simulink library "Displays_Lib"  (Simulink 8.1)
settings: Solver=ode45  StartTime=0.0  StopTime=10.0  RelTol=1e-3
undefined symbols (not defined in the file): ending_column_index, ending_row_index, framebuffer_16x1, framebuffer_2x2, framebuffer_4x4, framebuffer_8x8, HEIGHT, hot, POS_X, POS_Y, starting_column_index, starting_row_index, WIDTH
libraries: dspmtrx3 x119, commutil2 x100, dspsnks4 x4
(part 2 of 2)

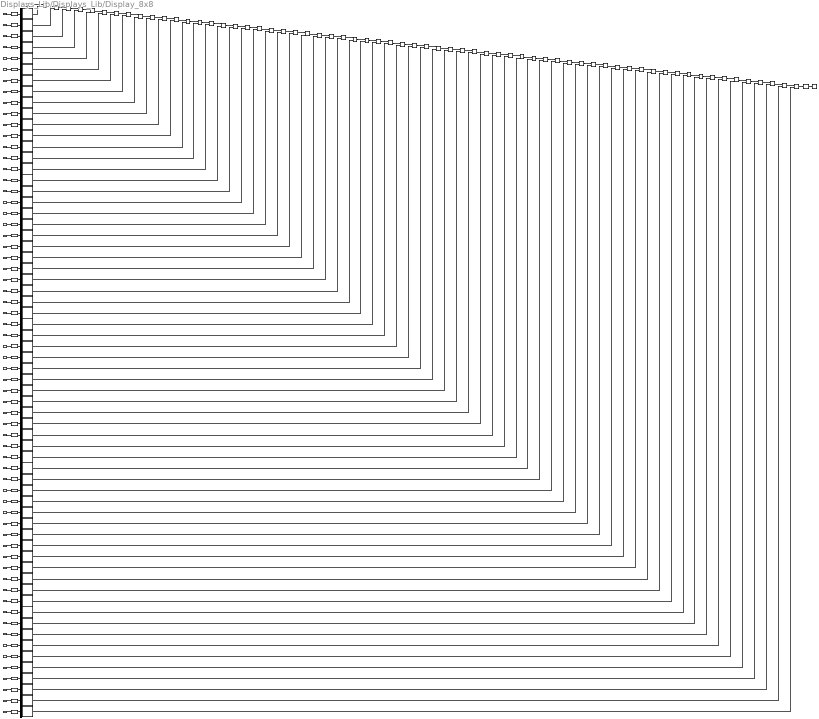
== system Displays_Lib/Displays_Lib/Display_8x8 ==
  Row1_Col1(8x1B) : Inport
  Row1_Col2(8x1B) : Inport  Port=2
  Row1_Col3(8x1B) : Inport  Port=3
  Row1_Col4(8x1B) : Inport  Port=4
  Row1_Col5(8x1B) : Inport  Port=5
  Row1_Col6(8x1B) : Inport  Port=6
  Row1_Col7(8x1B) : Inport  Port=7
  Row1_Col8(8x1B) : Inport  Port=8
  Row2_Col1(8x1B) : Inport  Port=9
  Row2_Col2(8x1B) : Inport  Port=10
  Row2_Col3(8x1B) : Inport  Port=11
  Row2_Col4(8x1B) : Inport  Port=12
  Row2_Col5(8x1B) : Inport  Port=13
  Row2_Col6(8x1B) : Inport  Port=14
  Row2_Col7(8x1B) : Inport  Port=15
  Row2_Col8(8x1B) : Inport  Port=16
  Row3_Col1(8x1B) : Inport  Port=17
  Row3_Col2(8x1B) : Inport  Port=18
  Row3_Col3(8x1B) : Inport  Port=19
  Row3_Col4(8x1B) : Inport  Port=20
  Row3_Col5(8x1B) : Inport  Port=21
  Row3_Col6(8x1B) : Inport  Port=22
  Row3_Col7(8x1B) : Inport  Port=23
  Row3_Col8(8x1B) : Inport  Port=24
  Row4_Col1(8x1B) : Inport  Port=25
  Row4_Col2(8x1B) : Inport  Port=26
  Row4_Col3(8x1B) : Inport  Port=27
  Row4_Col4(8x1B) : Inport  Port=28
  Row4_Col5(8x1B) : Inport  Port=29
  Row4_Col6(8x1B) : Inport  Port=30
  Row4_Col7(8x1B) : Inport  Port=31
  Row4_Col8(8x1B) : Inport  Port=32
  Row5_Col1(8x1B) : Inport  Port=33
  Row5_Col2(8x1B) : Inport  Port=34
  Row5_Col3(8x1B) : Inport  Port=35
  Row5_Col4(8x1B) : Inport  Port=36
  Row5_Col5(8x1B) : Inport  Port=37
  Row5_Col6(8x1B) : Inport  Port=38
  Row5_Col7(8x1B) : Inport  Port=39
  Row5_Col8(8x1B) : Inport  Port=40
  Row6_Col1(8x1B) : Inport  Port=41
  Row6_Col2(8x1B) : Inport  Port=42
  Row6_Col3(8x1B) : Inport  Port=43
  Row6_Col4(8x1B) : Inport  Port=44
  Row6_Col5(8x1B) : Inport  Port=45
  Row6_Col6(8x1B) : Inport  Port=46
  Row6_Col7(8x1B) : Inport  Port=47
  Row6_Col8(8x1B) : Inport  Port=48
  Row7_Col1(8x1B) : Inport  Port=49
  Row7_Col2(8x1B) : Inport  Port=50
  Row7_Col3(8x1B) : Inport  Port=51
  Row7_Col4(8x1B) : Inport  Port=52
  Row7_Col5(8x1B) : Inport  Port=53
  Row7_Col6(8x1B) : Inport  Port=54
  Row7_Col7(8x1B) : Inport  Port=55
  Row7_Col8(8x1B) : Inport  Port=56
  Row8_Col1(8x1B) : Inport  Port=57
  Row8_Col2(8x1B) : Inport  Port=58
  Row8_Col3(8x1B) : Inport  Port=59
  Row8_Col4(8x1B) : Inport  Port=60
  Row8_Col5(8x1B) : Inport  Port=61
  Row8_Col6(8x1B) : Inport  Port=62
  Row8_Col7(8x1B) : Inport  Port=63
  Row8_Col8(8x1B) : Inport  Port=64
  Constant1 : Constant  Value=framebuffer_8x8  OutDataTypeStr=uint8
  Demux{1..3,20..80} (64 alike) : Demux  Outputs=8
  Integer to Bit Converter{1..3,17,21..80} (64 alike) : commutil2/Integer to Bit Converter  nbits=8  signedInputValues=Unsigned  bitOrder=MSB first  outDtype=uint8
  Matrix Concatenate{1..4,21..80} (64 alike) : Concatenate  NumInputs=8  Mode=Multidimensional array  ConcatenateDimension=2
  Matrix Viewer3 : dspsnks4/Matrix Viewer  ImageParams=off  CMapStr=hot(256)  AxisColorbar=on  AxisParams=off  AxisOrigin=Upper left corner  XLabel=X-axis  YLabel=Y-axis  ZLabel=Z-axis  FigPos=[POS_X POS_Y-140 WIDTH HEIGHT]  AxisZoom=on
      settings: YMin=0  YMax=1.0
  Overwrite Values1 : dspmtrx3/Overwrite Values  OverWriteDiag=Submatrix  valFrom2ndIP=Second input port  ConstValue=0  RowSpan=Range of rows  RowStartMode=Index  RowStartIndex=starting_row_index(3)  RowEndMode=Index  RowEndIndex=ending_row_index(3)  ColSpan=Range of columns  ColStartMode=Index  ColStartIndex=starting_column_index(2)  ColEndMode=Index  ColEndIndex=ending_column_index(2)  DiagSpan=Range of elements  DiagStartMode=Index  DiagStartIndex=2  DiagEndMode=Index  DiagEndIndex=4
  Overwrite Values15 : dspmtrx3/Overwrite Values  OverWriteDiag=Submatrix  valFrom2ndIP=Second input port  ConstValue=0  RowSpan=Range of rows  RowStartMode=Index  RowStartIndex=starting_row_index(3)  RowEndMode=Index  RowEndIndex=ending_row_index(3)  ColSpan=Range of columns  ColStartMode=Index  ColStartIndex=starting_column_index(4)  ColEndMode=Index  ColEndIndex=ending_column_index(4)  DiagSpan=Range of elements  DiagStartMode=Index  DiagStartIndex=2  DiagEndMode=Index  DiagEndIndex=4
  Overwrite Values17 : dspmtrx3/Overwrite Values  OverWriteDiag=Submatrix  valFrom2ndIP=Second input port  ConstValue=0  RowSpan=Range of rows  RowStartMode=Index  RowStartIndex=starting_row_index(3)  RowEndMode=Index  RowEndIndex=ending_row_index(3)  ColSpan=Range of columns  ColStartMode=Index  ColStartIndex=starting_column_index(1)  ColEndMode=Index  ColEndIndex=ending_column_index(1)  DiagSpan=Range of elements  DiagStartMode=Index  DiagStartIndex=2  DiagEndMode=Index  DiagEndIndex=4
  Overwrite Values18 : dspmtrx3/Overwrite Values  OverWriteDiag=Submatrix  valFrom2ndIP=Second input port  ConstValue=0  RowSpan=Range of rows  RowStartMode=Index  RowStartIndex=starting_row_index(5)  RowEndMode=Index  RowEndIndex=ending_row_index(5)  ColSpan=Range of columns  ColStartMode=Index  ColStartIndex=starting_column_index(2)  ColEndMode=Index  ColEndIndex=ending_column_index(2)  DiagSpan=Range of elements  DiagStartMode=Index  DiagStartIndex=2  DiagEndMode=Index  DiagEndIndex=4
  Overwrite Values19 : dspmtrx3/Overwrite Values  OverWriteDiag=Submatrix  valFrom2ndIP=Second input port  ConstValue=0  RowSpan=Range of rows  RowStartMode=Index  RowStartIndex=starting_row_index(4)  RowEndMode=Index  RowEndIndex=ending_row_index(4)  ColSpan=Range of columns  ColStartMode=Index  ColStartIndex=starting_column_index(4)  ColEndMode=Index  ColEndIndex=ending_column_index(4)  DiagSpan=Range of elements  DiagStartMode=Index  DiagStartIndex=2  DiagEndMode=Index  DiagEndIndex=4
  Overwrite Values2 : dspmtrx3/Overwrite Values  OverWriteDiag=Submatrix  valFrom2ndIP=Second input port  ConstValue=0  RowSpan=Range of rows  RowStartMode=Index  RowStartIndex=starting_row_index(8)  RowEndMode=Index  RowEndIndex=ending_row_index(8)  ColSpan=Range of columns  ColStartMode=Index  ColStartIndex=starting_column_index(3)  ColEndMode=Index  ColEndIndex=ending_column_index(3)  DiagSpan=Range of elements  DiagStartMode=Index  DiagStartIndex=2  DiagEndMode=Index  DiagEndIndex=4
  Overwrite Values21 : dspmtrx3/Overwrite Values  OverWriteDiag=Submatrix  valFrom2ndIP=Second input port  ConstValue=0  RowSpan=Range of rows  RowStartMode=Index  RowStartIndex=starting_row_index(5)  RowEndMode=Index  RowEndIndex=ending_row_index(5)  ColSpan=Range of columns  ColStartMode=Index  ColStartIndex=starting_column_index(4)  ColEndMode=Index  ColEndIndex=ending_column_index(4)  DiagSpan=Range of elements  DiagStartMode=Index  DiagStartIndex=2  DiagEndMode=Index  DiagEndIndex=4
  Overwrite Values22 : dspmtrx3/Overwrite Values  OverWriteDiag=Submatrix  valFrom2ndIP=Second input port  ConstValue=0  RowSpan=Range of rows  RowStartMode=Index  RowStartIndex=starting_row_index(6)  RowEndMode=Index  RowEndIndex=ending_row_index(6)  ColSpan=Range of columns  ColStartMode=Index  ColStartIndex=starting_column_index(4)  ColEndMode=Index  ColEndIndex=ending_column_index(4)  DiagSpan=Range of elements  DiagStartMode=Index  DiagStartIndex=2  DiagEndMode=Index  DiagEndIndex=4
  Overwrite Values25 : dspmtrx3/Overwrite Values  OverWriteDiag=Submatrix  valFrom2ndIP=Second input port  ConstValue=0  RowSpan=Range of rows  RowStartMode=Index  RowStartIndex=starting_row_index(7)  RowEndMode=Index  RowEndIndex=ending_row_index(7)  ColSpan=Range of columns  ColStartMode=Index  ColStartIndex=starting_column_index(4)  ColEndMode=Index  ColEndIndex=ending_column_index(4)  DiagSpan=Range of elements  DiagStartMode=Index  DiagStartIndex=2  DiagEndMode=Index  DiagEndIndex=4
  Overwrite Values26 : dspmtrx3/Overwrite Values  OverWriteDiag=Submatrix  valFrom2ndIP=Second input port  ConstValue=0  RowSpan=Range of rows  RowStartMode=Index  RowStartIndex=starting_row_index(3)  RowEndMode=Index  RowEndIndex=ending_row_index(3)  ColSpan=Range of columns  ColStartMode=Index  ColStartIndex=starting_column_index(3)  ColEndMode=Index  ColEndIndex=ending_column_index(3)  DiagSpan=Range of elements  DiagStartMode=Index  DiagStartIndex=2  DiagEndMode=Index  DiagEndIndex=4
  Overwrite Values27 : dspmtrx3/Overwrite Values  OverWriteDiag=Submatrix  valFrom2ndIP=Second input port  ConstValue=0  RowSpan=Range of rows  RowStartMode=Index  RowStartIndex=starting_row_index(4)  RowEndMode=Index  RowEndIndex=ending_row_index(4)  ColSpan=Range of columns  ColStartMode=Index  ColStartIndex=starting_column_index(1)  ColEndMode=Index  ColEndIndex=ending_column_index(1)  DiagSpan=Range of elements  DiagStartMode=Index  DiagStartIndex=2  DiagEndMode=Index  DiagEndIndex=4
  Overwrite Values28 : dspmtrx3/Overwrite Values  OverWriteDiag=Submatrix  valFrom2ndIP=Second input port  ConstValue=0  RowSpan=Range of rows  RowStartMode=Index  RowStartIndex=starting_row_index(6)  RowEndMode=Index  RowEndIndex=ending_row_index(6)  ColSpan=Range of columns  ColStartMode=Index  ColStartIndex=starting_column_index(2)  ColEndMode=Index  ColEndIndex=ending_column_index(2)  DiagSpan=Range of elements  DiagStartMode=Index  DiagStartIndex=2  DiagEndMode=Index  DiagEndIndex=4
  Overwrite Values29 : dspmtrx3/Overwrite Values  OverWriteDiag=Submatrix  valFrom2ndIP=Second input port  ConstValue=0  RowSpan=Range of rows  RowStartMode=Index  RowStartIndex=starting_row_index(8)  RowEndMode=Index  RowEndIndex=ending_row_index(8)  ColSpan=Range of columns  ColStartMode=Index  ColStartIndex=starting_column_index(4)  ColEndMode=Index  ColEndIndex=ending_column_index(4)  DiagSpan=Range of elements  DiagStartMode=Index  DiagStartIndex=2  DiagEndMode=Index  DiagEndIndex=4
  Overwrite Values3 : dspmtrx3/Overwrite Values  OverWriteDiag=Submatrix  valFrom2ndIP=Second input port  ConstValue=0  RowSpan=Range of rows  RowStartMode=Index  RowStartIndex=starting_row_index(1)  RowEndMode=Index  RowEndIndex=ending_row_index(1)  ColSpan=Range of columns  ColStartMode=Index  ColStartIndex=starting_column_index(3)  ColEndMode=Index  ColEndIndex=ending_column_index(3)  DiagSpan=Range of elements  DiagStartMode=Index  DiagStartIndex=2  DiagEndMode=Index  DiagEndIndex=4
  Overwrite Values30 : dspmtrx3/Overwrite Values  OverWriteDiag=Submatrix  valFrom2ndIP=Second input port  ConstValue=0  RowSpan=Range of rows  RowStartMode=Index  RowStartIndex=starting_row_index(1)  RowEndMode=Index  RowEndIndex=ending_row_index(1)  ColSpan=Range of columns  ColStartMode=Index  ColStartIndex=starting_column_index(4)  ColEndMode=Index  ColEndIndex=ending_column_index(4)  DiagSpan=Range of elements  DiagStartMode=Index  DiagStartIndex=2  DiagEndMode=Index  DiagEndIndex=4
  Overwrite Values31 : dspmtrx3/Overwrite Values  OverWriteDiag=Submatrix  valFrom2ndIP=Second input port  ConstValue=0  RowSpan=Range of rows  RowStartMode=Index  RowStartIndex=starting_row_index(2)  RowEndMode=Index  RowEndIndex=ending_row_index(2)  ColSpan=Range of columns  ColStartMode=Index  ColStartIndex=starting_column_index(4)  ColEndMode=Index  ColEndIndex=ending_column_index(4)  DiagSpan=Range of elements  DiagStartMode=Index  DiagStartIndex=2  DiagEndMode=Index  DiagEndIndex=4
  Overwrite Values32 : dspmtrx3/Overwrite Values  OverWriteDiag=Submatrix  valFrom2ndIP=Second input port  ConstValue=0  RowSpan=Range of rows  RowStartMode=Index  RowStartIndex=starting_row_index(3)  RowEndMode=Index  RowEndIndex=ending_row_index(3)  ColSpan=Range of columns  ColStartMode=Index  ColStartIndex=starting_column_index(5)  ColEndMode=Index  ColEndIndex=ending_column_index(5)  DiagSpan=Range of elements  DiagStartMode=Index  DiagStartIndex=2  DiagEndMode=Index  DiagEndIndex=4
  Overwrite Values33 : dspmtrx3/Overwrite Values  OverWriteDiag=Submatrix  valFrom2ndIP=Second input port  ConstValue=0  RowSpan=Range of rows  RowStartMode=Index  RowStartIndex=starting_row_index(5)  RowEndMode=Index  RowEndIndex=ending_row_index(5)  ColSpan=Range of columns  ColStartMode=Index  ColStartIndex=starting_column_index(1)  ColEndMode=Index  ColEndIndex=ending_column_index(1)  DiagSpan=Range of elements  DiagStartMode=Index  DiagStartIndex=2  DiagEndMode=Index  DiagEndIndex=4
  Overwrite Values34 : dspmtrx3/Overwrite Values  OverWriteDiag=Submatrix  valFrom2ndIP=Second input port  ConstValue=0  RowSpan=Range of rows  RowStartMode=Index  RowStartIndex=starting_row_index(7)  RowEndMode=Index  RowEndIndex=ending_row_index(7)  ColSpan=Range of columns  ColStartMode=Index  ColStartIndex=starting_column_index(2)  ColEndMode=Index  ColEndIndex=ending_column_index(2)  DiagSpan=Range of elements  DiagStartMode=Index  DiagStartIndex=2  DiagEndMode=Index  DiagEndIndex=4
  Overwrite Values35 : dspmtrx3/Overwrite Values  OverWriteDiag=Submatrix  valFrom2ndIP=Second input port  ConstValue=0  RowSpan=Range of rows  RowStartMode=Index  RowStartIndex=starting_row_index(4)  RowEndMode=Index  RowEndIndex=ending_row_index(4)  ColSpan=Range of columns  ColStartMode=Index  ColStartIndex=starting_column_index(5)  ColEndMode=Index  ColEndIndex=ending_column_index(5)  DiagSpan=Range of elements  DiagStartMode=Index  DiagStartIndex=2  DiagEndMode=Index  DiagEndIndex=4
  Overwrite Values36 : dspmtrx3/Overwrite Values  OverWriteDiag=Submatrix  valFrom2ndIP=Second input port  ConstValue=0  RowSpan=Range of rows  RowStartMode=Index  RowStartIndex=starting_row_index(5)  RowEndMode=Index  RowEndIndex=ending_row_index(5)  ColSpan=Range of columns  ColStartMode=Index  ColStartIndex=starting_column_index(5)  ColEndMode=Index  ColEndIndex=ending_column_index(5)  DiagSpan=Range of elements  DiagStartMode=Index  DiagStartIndex=2  DiagEndMode=Index  DiagEndIndex=4
  Overwrite Values39 : dspmtrx3/Overwrite Values  OverWriteDiag=Submatrix  valFrom2ndIP=Second input port  ConstValue=0  RowSpan=Range of rows  RowStartMode=Index  RowStartIndex=starting_row_index(4)  RowEndMode=Index  RowEndIndex=ending_row_index(4)  ColSpan=Range of columns  ColStartMode=Index  ColStartIndex=starting_column_index(3)  ColEndMode=Index  ColEndIndex=ending_column_index(3)  DiagSpan=Range of elements  DiagStartMode=Index  DiagStartIndex=2  DiagEndMode=Index  DiagEndIndex=4
  Overwrite Values4 : dspmtrx3/Overwrite Values  OverWriteDiag=Submatrix  valFrom2ndIP=Second input port  ConstValue=0  RowSpan=Range of rows  RowStartMode=Index  RowStartIndex=starting_row_index(2)  RowEndMode=Index  RowEndIndex=ending_row_index(2)  ColSpan=Range of columns  ColStartMode=Index  ColStartIndex=starting_column_index(3)  ColEndMode=Index  ColEndIndex=ending_column_index(3)  DiagSpan=Range of elements  DiagStartMode=Index  DiagStartIndex=2  DiagEndMode=Index  DiagEndIndex=4
  Overwrite Values40 : dspmtrx3/Overwrite Values  OverWriteDiag=Submatrix  valFrom2ndIP=Second input port  ConstValue=0  RowSpan=Range of rows  RowStartMode=Index  RowStartIndex=starting_row_index(6)  RowEndMode=Index  RowEndIndex=ending_row_index(6)  ColSpan=Range of columns  ColStartMode=Index  ColStartIndex=starting_column_index(5)  ColEndMode=Index  ColEndIndex=ending_column_index(5)  DiagSpan=Range of elements  DiagStartMode=Index  DiagStartIndex=2  DiagEndMode=Index  DiagEndIndex=4
  Overwrite Values41 : dspmtrx3/Overwrite Values  OverWriteDiag=Submatrix  valFrom2ndIP=Second input port  ConstValue=0  RowSpan=Range of rows  RowStartMode=Index  RowStartIndex=starting_row_index(7)  RowEndMode=Index  RowEndIndex=ending_row_index(7)  ColSpan=Range of columns  ColStartMode=Index  ColStartIndex=starting_column_index(5)  ColEndMode=Index  ColEndIndex=ending_column_index(5)  DiagSpan=Range of elements  DiagStartMode=Index  DiagStartIndex=2  DiagEndMode=Index  DiagEndIndex=4
  Overwrite Values42 : dspmtrx3/Overwrite Values  OverWriteDiag=Submatrix  valFrom2ndIP=Second input port  ConstValue=0  RowSpan=Range of rows  RowStartMode=Index  RowStartIndex=starting_row_index(6)  RowEndMode=Index  RowEndIndex=ending_row_index(6)  ColSpan=Range of columns  ColStartMode=Index  ColStartIndex=starting_column_index(1)  ColEndMode=Index  ColEndIndex=ending_column_index(1)  DiagSpan=Range of elements  DiagStartMode=Index  DiagStartIndex=2  DiagEndMode=Index  DiagEndIndex=4
  Overwrite Values43 : dspmtrx3/Overwrite Values  OverWriteDiag=Submatrix  valFrom2ndIP=Second input port  ConstValue=0  RowSpan=Range of rows  RowStartMode=Index  RowStartIndex=starting_row_index(8)  RowEndMode=Index  RowEndIndex=ending_row_index(8)  ColSpan=Range of columns  ColStartMode=Index  ColStartIndex=starting_column_index(2)  ColEndMode=Index  ColEndIndex=ending_column_index(2)  DiagSpan=Range of elements  DiagStartMode=Index  DiagStartIndex=2  DiagEndMode=Index  DiagEndIndex=4
  Overwrite Values44 : dspmtrx3/Overwrite Values  OverWriteDiag=Submatrix  valFrom2ndIP=Second input port  ConstValue=0  RowSpan=Range of rows  RowStartMode=Index  RowStartIndex=starting_row_index(8)  RowEndMode=Index  RowEndIndex=ending_row_index(8)  ColSpan=Range of columns  ColStartMode=Index  ColStartIndex=starting_column_index(5)  ColEndMode=Index  ColEndIndex=ending_column_index(5)  DiagSpan=Range of elements  DiagStartMode=Index  DiagStartIndex=2  DiagEndMode=Index  DiagEndIndex=4
  Overwrite Values45 : dspmtrx3/Overwrite Values  OverWriteDiag=Submatrix  valFrom2ndIP=Second input port  ConstValue=0  RowSpan=Range of rows  RowStartMode=Index  RowStartIndex=starting_row_index(7)  RowEndMode=Index  RowEndIndex=ending_row_index(7)  ColSpan=Range of columns  ColStartMode=Index  ColStartIndex=starting_column_index(1)  ColEndMode=Index  ColEndIndex=ending_column_index(1)  DiagSpan=Range of elements  DiagStartMode=Index  DiagStartIndex=2  DiagEndMode=Index  DiagEndIndex=4
  Overwrite Values46 : dspmtrx3/Overwrite Values  OverWriteDiag=Submatrix  valFrom2ndIP=Second input port  ConstValue=0  RowSpan=Range of rows  RowStartMode=Index  RowStartIndex=starting_row_index(8)  RowEndMode=Index  RowEndIndex=ending_row_index(8)  ColSpan=Range of columns  ColStartMode=Index  ColStartIndex=starting_column_index(1)  ColEndMode=Index  ColEndIndex=ending_column_index(1)  DiagSpan=Range of elements  DiagStartMode=Index  DiagStartIndex=2  DiagEndMode=Index  DiagEndIndex=4
  Overwrite Values47 : dspmtrx3/Overwrite Values  OverWriteDiag=Submatrix  valFrom2ndIP=Second input port  ConstValue=0  RowSpan=Range of rows  RowStartMode=Index  RowStartIndex=starting_row_index(1)  RowEndMode=Index  RowEndIndex=ending_row_index(1)  ColSpan=Range of columns  ColStartMode=Index  ColStartIndex=starting_column_index(2)  ColEndMode=Index  ColEndIndex=ending_column_index(2)  DiagSpan=Range of elements  DiagStartMode=Index  DiagStartIndex=2  DiagEndMode=Index  DiagEndIndex=4
  Overwrite Values48 : dspmtrx3/Overwrite Values  OverWriteDiag=Submatrix  valFrom2ndIP=Second input port  ConstValue=0  RowSpan=Range of rows  RowStartMode=Index  RowStartIndex=starting_row_index(2)  RowEndMode=Index  RowEndIndex=ending_row_index(2)  ColSpan=Range of columns  ColStartMode=Index  ColStartIndex=starting_column_index(2)  ColEndMode=Index  ColEndIndex=ending_column_index(2)  DiagSpan=Range of elements  DiagStartMode=Index  DiagStartIndex=2  DiagEndMode=Index  DiagEndIndex=4
  Overwrite Values49 : dspmtrx3/Overwrite Values  OverWriteDiag=Submatrix  valFrom2ndIP=Second input port  ConstValue=0  RowSpan=Range of rows  RowStartMode=Index  RowStartIndex=starting_row_index(1)  RowEndMode=Index  RowEndIndex=ending_row_index(1)  ColSpan=Range of columns  ColStartMode=Index  ColStartIndex=starting_column_index(5)  ColEndMode=Index  ColEndIndex=ending_column_index(5)  DiagSpan=Range of elements  DiagStartMode=Index  DiagStartIndex=2  DiagEndMode=Index  DiagEndIndex=4
  Overwrite Values50 : dspmtrx3/Overwrite Values  OverWriteDiag=Submatrix  valFrom2ndIP=Second input port  ConstValue=0  RowSpan=Range of rows  RowStartMode=Index  RowStartIndex=starting_row_index(5)  RowEndMode=Index  RowEndIndex=ending_row_index(5)  ColSpan=Range of columns  ColStartMode=Index  ColStartIndex=starting_column_index(3)  ColEndMode=Index  ColEndIndex=ending_column_index(3)  DiagSpan=Range of elements  DiagStartMode=Index  DiagStartIndex=2  DiagEndMode=Index  DiagEndIndex=4
  Overwrite Values51 : dspmtrx3/Overwrite Values  OverWriteDiag=Submatrix  valFrom2ndIP=Second input port  ConstValue=0  RowSpan=Range of rows  RowStartMode=Index  RowStartIndex=starting_row_index(2)  RowEndMode=Index  RowEndIndex=ending_row_index(2)  ColSpan=Range of columns  ColStartMode=Index  ColStartIndex=starting_column_index(5)  ColEndMode=Index  ColEndIndex=ending_column_index(5)  DiagSpan=Range of elements  DiagStartMode=Index  DiagStartIndex=2  DiagEndMode=Index  DiagEndIndex=4
  Overwrite Values52 : dspmtrx3/Overwrite Values  OverWriteDiag=Submatrix  valFrom2ndIP=Second input port  ConstValue=0  RowSpan=Range of rows  RowStartMode=Index  RowStartIndex=starting_row_index(3)  RowEndMode=Index  RowEndIndex=ending_row_index(3)  ColSpan=Range of columns  ColStartMode=Index  ColStartIndex=starting_column_index(6)  ColEndMode=Index  ColEndIndex=ending_column_index(6)  DiagSpan=Range of elements  DiagStartMode=Index  DiagStartIndex=2  DiagEndMode=Index  DiagEndIndex=4
  Overwrite Values53 : dspmtrx3/Overwrite Values  OverWriteDiag=Submatrix  valFrom2ndIP=Second input port  ConstValue=0  RowSpan=Range of rows  RowStartMode=Index  RowStartIndex=starting_row_index(4)  RowEndMode=Index  RowEndIndex=ending_row_index(4)  ColSpan=Range of columns  ColStartMode=Index  ColStartIndex=starting_column_index(6)  ColEndMode=Index  ColEndIndex=ending_column_index(6)  DiagSpan=Range of elements  DiagStartMode=Index  DiagStartIndex=2  DiagEndMode=Index  DiagEndIndex=4
  Overwrite Values54 : dspmtrx3/Overwrite Values  OverWriteDiag=Submatrix  valFrom2ndIP=Second input port  ConstValue=0  RowSpan=Range of rows  RowStartMode=Index  RowStartIndex=starting_row_index(5)  RowEndMode=Index  RowEndIndex=ending_row_index(5)  ColSpan=Range of columns  ColStartMode=Index  ColStartIndex=starting_column_index(6)  ColEndMode=Index  ColEndIndex=ending_column_index(6)  DiagSpan=Range of elements  DiagStartMode=Index  DiagStartIndex=2  DiagEndMode=Index  DiagEndIndex=4
  Overwrite Values55 : dspmtrx3/Overwrite Values  OverWriteDiag=Submatrix  valFrom2ndIP=Second input port  ConstValue=0  RowSpan=Range of rows  RowStartMode=Index  RowStartIndex=starting_row_index(6)  RowEndMode=Index  RowEndIndex=ending_row_index(6)  ColSpan=Range of columns  ColStartMode=Index  ColStartIndex=starting_column_index(6)  ColEndMode=Index  ColEndIndex=ending_column_index(6)  DiagSpan=Range of elements  DiagStartMode=Index  DiagStartIndex=2  DiagEndMode=Index  DiagEndIndex=4
  Overwrite Values56 : dspmtrx3/Overwrite Values  OverWriteDiag=Submatrix  valFrom2ndIP=Second input port  ConstValue=0  RowSpan=Range of rows  RowStartMode=Index  RowStartIndex=starting_row_index(7)  RowEndMode=Index  RowEndIndex=ending_row_index(7)  ColSpan=Range of columns  ColStartMode=Index  ColStartIndex=starting_column_index(6)  ColEndMode=Index  ColEndIndex=ending_column_index(6)  DiagSpan=Range of elements  DiagStartMode=Index  DiagStartIndex=2  DiagEndMode=Index  DiagEndIndex=4
  Overwrite Values57 : dspmtrx3/Overwrite Values  OverWriteDiag=Submatrix  valFrom2ndIP=Second input port  ConstValue=0  RowSpan=Range of rows  RowStartMode=Index  RowStartIndex=starting_row_index(8)  RowEndMode=Index  RowEndIndex=ending_row_index(8)  ColSpan=Range of columns  ColStartMode=Index  ColStartIndex=starting_column_index(6)  ColEndMode=Index  ColEndIndex=ending_column_index(6)  DiagSpan=Range of elements  DiagStartMode=Index  DiagStartIndex=2  DiagEndMode=Index  DiagEndIndex=4
  Overwrite Values58 : dspmtrx3/Overwrite Values  OverWriteDiag=Submatrix  valFrom2ndIP=Second input port  ConstValue=0  RowSpan=Range of rows  RowStartMode=Index  RowStartIndex=starting_row_index(1)  RowEndMode=Index  RowEndIndex=ending_row_index(1)  ColSpan=Range of columns  ColStartMode=Index  ColStartIndex=starting_column_index(6)  ColEndMode=Index  ColEndIndex=ending_column_index(6)  DiagSpan=Range of elements  DiagStartMode=Index  DiagStartIndex=2  DiagEndMode=Index  DiagEndIndex=4
  Overwrite Values59 : dspmtrx3/Overwrite Values  OverWriteDiag=Submatrix  valFrom2ndIP=Second input port  ConstValue=0  RowSpan=Range of rows  RowStartMode=Index  RowStartIndex=starting_row_index(2)  RowEndMode=Index  RowEndIndex=ending_row_index(2)  ColSpan=Range of columns  ColStartMode=Index  ColStartIndex=starting_column_index(6)  ColEndMode=Index  ColEndIndex=ending_column_index(6)  DiagSpan=Range of elements  DiagStartMode=Index  DiagStartIndex=2  DiagEndMode=Index  DiagEndIndex=4
  Overwrite Values60 : dspmtrx3/Overwrite Values  OverWriteDiag=Submatrix  valFrom2ndIP=Second input port  ConstValue=0  RowSpan=Range of rows  RowStartMode=Index  RowStartIndex=starting_row_index(3)  RowEndMode=Index  RowEndIndex=ending_row_index(3)  ColSpan=Range of columns  ColStartMode=Index  ColStartIndex=starting_column_index(7)  ColEndMode=Index  ColEndIndex=ending_column_index(7)  DiagSpan=Range of elements  DiagStartMode=Index  DiagStartIndex=2  DiagEndMode=Index  DiagEndIndex=4
  Overwrite Values61 : dspmtrx3/Overwrite Values  OverWriteDiag=Submatrix  valFrom2ndIP=Second input port  ConstValue=0  RowSpan=Range of rows  RowStartMode=Index  RowStartIndex=starting_row_index(6)  RowEndMode=Index  RowEndIndex=ending_row_index(6)  ColSpan=Range of columns  ColStartMode=Index  ColStartIndex=starting_column_index(3)  ColEndMode=Index  ColEndIndex=ending_column_index(3)  DiagSpan=Range of elements  DiagStartMode=Index  DiagStartIndex=2  DiagEndMode=Index  DiagEndIndex=4
  Overwrite Values62 : dspmtrx3/Overwrite Values  OverWriteDiag=Submatrix  valFrom2ndIP=Second input port  ConstValue=0  RowSpan=Range of rows  RowStartMode=Index  RowStartIndex=starting_row_index(4)  RowEndMode=Index  RowEndIndex=ending_row_index(4)  ColSpan=Range of columns  ColStartMode=Index  ColStartIndex=starting_column_index(7)  ColEndMode=Index  ColEndIndex=ending_column_index(7)  DiagSpan=Range of elements  DiagStartMode=Index  DiagStartIndex=2  DiagEndMode=Index  DiagEndIndex=4
  Overwrite Values63 : dspmtrx3/Overwrite Values  OverWriteDiag=Submatrix  valFrom2ndIP=Second input port  ConstValue=0  RowSpan=Range of rows  RowStartMode=Index  RowStartIndex=starting_row_index(5)  RowEndMode=Index  RowEndIndex=ending_row_index(5)  ColSpan=Range of columns  ColStartMode=Index  ColStartIndex=starting_column_index(7)  ColEndMode=Index  ColEndIndex=ending_column_index(7)  DiagSpan=Range of elements  DiagStartMode=Index  DiagStartIndex=2  DiagEndMode=Index  DiagEndIndex=4
  Overwrite Values64 : dspmtrx3/Overwrite Values  OverWriteDiag=Submatrix  valFrom2ndIP=Second input port  ConstValue=0  RowSpan=Range of rows  RowStartMode=Index  RowStartIndex=starting_row_index(6)  RowEndMode=Index  RowEndIndex=ending_row_index(6)  ColSpan=Range of columns  ColStartMode=Index  ColStartIndex=starting_column_index(7)  ColEndMode=Index  ColEndIndex=ending_column_index(7)  DiagSpan=Range of elements  DiagStartMode=Index  DiagStartIndex=2  DiagEndMode=Index  DiagEndIndex=4
  Overwrite Values65 : dspmtrx3/Overwrite Values  OverWriteDiag=Submatrix  valFrom2ndIP=Second input port  ConstValue=0  RowSpan=Range of rows  RowStartMode=Index  RowStartIndex=starting_row_index(7)  RowEndMode=Index  RowEndIndex=ending_row_index(7)  ColSpan=Range of columns  ColStartMode=Index  ColStartIndex=starting_column_index(7)  ColEndMode=Index  ColEndIndex=ending_column_index(7)  DiagSpan=Range of elements  DiagStartMode=Index  DiagStartIndex=2  DiagEndMode=Index  DiagEndIndex=4
  Overwrite Values66 : dspmtrx3/Overwrite Values  OverWriteDiag=Submatrix  valFrom2ndIP=Second input port  ConstValue=0  RowSpan=Range of rows  RowStartMode=Index  RowStartIndex=starting_row_index(8)  RowEndMode=Index  RowEndIndex=ending_row_index(8)  ColSpan=Range of columns  ColStartMode=Index  ColStartIndex=starting_column_index(7)  ColEndMode=Index  ColEndIndex=ending_column_index(7)  DiagSpan=Range of elements  DiagStartMode=Index  DiagStartIndex=2  DiagEndMode=Index  DiagEndIndex=4
  Overwrite Values67 : dspmtrx3/Overwrite Values  OverWriteDiag=Submatrix  valFrom2ndIP=Second input port  ConstValue=0  RowSpan=Range of rows  RowStartMode=Index  RowStartIndex=starting_row_index(1)  RowEndMode=Index  RowEndIndex=ending_row_index(1)  ColSpan=Range of columns  ColStartMode=Index  ColStartIndex=starting_column_index(7)  ColEndMode=Index  ColEndIndex=ending_column_index(7)  DiagSpan=Range of elements  DiagStartMode=Index  DiagStartIndex=2  DiagEndMode=Index  DiagEndIndex=4
  Overwrite Values68 : dspmtrx3/Overwrite Values  OverWriteDiag=Submatrix  valFrom2ndIP=Second input port  ConstValue=0  RowSpan=Range of rows  RowStartMode=Index  RowStartIndex=starting_row_index(2)  RowEndMode=Index  RowEndIndex=ending_row_index(2)  ColSpan=Range of columns  ColStartMode=Index  ColStartIndex=starting_column_index(7)  ColEndMode=Index  ColEndIndex=ending_column_index(7)  DiagSpan=Range of elements  DiagStartMode=Index  DiagStartIndex=2  DiagEndMode=Index  DiagEndIndex=4
  Overwrite Values69 : dspmtrx3/Overwrite Values  OverWriteDiag=Submatrix  valFrom2ndIP=Second input port  ConstValue=0  RowSpan=Range of rows  RowStartMode=Index  RowStartIndex=starting_row_index(3)  RowEndMode=Index  RowEndIndex=ending_row_index(3)  ColSpan=Range of columns  ColStartMode=Index  ColStartIndex=starting_column_index(8)  ColEndMode=Index  ColEndIndex=ending_column_index(8)  DiagSpan=Range of elements  DiagStartMode=Index  DiagStartIndex=2  DiagEndMode=Index  DiagEndIndex=4
  Overwrite Values70 : dspmtrx3/Overwrite Values  OverWriteDiag=Submatrix  valFrom2ndIP=Second input port  ConstValue=0  RowSpan=Range of rows  RowStartMode=Index  RowStartIndex=starting_row_index(4)  RowEndMode=Index  RowEndIndex=ending_row_index(4)  ColSpan=Range of columns  ColStartMode=Index  ColStartIndex=starting_column_index(8)  ColEndMode=Index  ColEndIndex=ending_column_index(8)  DiagSpan=Range of elements  DiagStartMode=Index  DiagStartIndex=2  DiagEndMode=Index  DiagEndIndex=4
  Overwrite Values71 : dspmtrx3/Overwrite Values  OverWriteDiag=Submatrix  valFrom2ndIP=Second input port  ConstValue=0  RowSpan=Range of rows  RowStartMode=Index  RowStartIndex=starting_row_index(5)  RowEndMode=Index  RowEndIndex=ending_row_index(5)  ColSpan=Range of columns  ColStartMode=Index  ColStartIndex=starting_column_index(8)  ColEndMode=Index  ColEndIndex=ending_column_index(8)  DiagSpan=Range of elements  DiagStartMode=Index  DiagStartIndex=2  DiagEndMode=Index  DiagEndIndex=4
  Overwrite Values72 : dspmtrx3/Overwrite Values  OverWriteDiag=Submatrix  valFrom2ndIP=Second input port  ConstValue=0  RowSpan=Range of rows  RowStartMode=Index  RowStartIndex=starting_row_index(7)  RowEndMode=Index  RowEndIndex=ending_row_index(7)  ColSpan=Range of columns  ColStartMode=Index  ColStartIndex=starting_column_index(3)  ColEndMode=Index  ColEndIndex=ending_column_index(3)  DiagSpan=Range of elements  DiagStartMode=Index  DiagStartIndex=2  DiagEndMode=Index  DiagEndIndex=4
  Overwrite Values73 : dspmtrx3/Overwrite Values  OverWriteDiag=Submatrix  valFrom2ndIP=Second input port  ConstValue=0  RowSpan=Range of rows  RowStartMode=Index  RowStartIndex=starting_row_index(6)  RowEndMode=Index  RowEndIndex=ending_row_index(6)  ColSpan=Range of columns  ColStartMode=Index  ColStartIndex=starting_column_index(8)  ColEndMode=Index  ColEndIndex=ending_column_index(8)  DiagSpan=Range of elements  DiagStartMode=Index  DiagStartIndex=2  DiagEndMode=Index  DiagEndIndex=4
  Overwrite Values74 : dspmtrx3/Overwrite Values  OverWriteDiag=Submatrix  valFrom2ndIP=Second input port  ConstValue=0  RowSpan=Range of rows  RowStartMode=Index  RowStartIndex=starting_row_index(7)  RowEndMode=Index  RowEndIndex=ending_row_index(7)  ColSpan=Range of columns  ColStartMode=Index  ColStartIndex=starting_column_index(8)  ColEndMode=Index  ColEndIndex=ending_column_index(8)  DiagSpan=Range of elements  DiagStartMode=Index  DiagStartIndex=2  DiagEndMode=Index  DiagEndIndex=4
  Overwrite Values75 : dspmtrx3/Overwrite Values  OverWriteDiag=Submatrix  valFrom2ndIP=Second input port  ConstValue=0  RowSpan=Range of rows  RowStartMode=Index  RowStartIndex=starting_row_index(8)  RowEndMode=Index  RowEndIndex=ending_row_index(8)  ColSpan=Range of columns  ColStartMode=Index  ColStartIndex=starting_column_index(8)  ColEndMode=Index  ColEndIndex=ending_column_index(8)  DiagSpan=Range of elements  DiagStartMode=Index  DiagStartIndex=2  DiagEndMode=Index  DiagEndIndex=4
  Overwrite Values76 : dspmtrx3/Overwrite Values  OverWriteDiag=Submatrix  valFrom2ndIP=Second input port  ConstValue=0  RowSpan=Range of rows  RowStartMode=Index  RowStartIndex=starting_row_index(1)  RowEndMode=Index  RowEndIndex=ending_row_index(1)  ColSpan=Range of columns  ColStartMode=Index  ColStartIndex=starting_column_index(8)  ColEndMode=Index  ColEndIndex=ending_column_index(8)  DiagSpan=Range of elements  DiagStartMode=Index  DiagStartIndex=2  DiagEndMode=Index  DiagEndIndex=4
  Overwrite Values77 : dspmtrx3/Overwrite Values  OverWriteDiag=Submatrix  valFrom2ndIP=Second input port  ConstValue=0  RowSpan=Range of rows  RowStartMode=Index  RowStartIndex=starting_row_index(2)  RowEndMode=Index  RowEndIndex=ending_row_index(2)  ColSpan=Range of columns  ColStartMode=Index  ColStartIndex=starting_column_index(8)  ColEndMode=Index  ColEndIndex=ending_column_index(8)  DiagSpan=Range of elements  DiagStartMode=Index  DiagStartIndex=2  DiagEndMode=Index  DiagEndIndex=4
  Overwrite Values78 : dspmtrx3/Overwrite Values  OverWriteDiag=Submatrix  valFrom2ndIP=Second input port  ConstValue=0  RowSpan=Range of rows  RowStartMode=Index  RowStartIndex=starting_row_index(1)  RowEndMode=Index  RowEndIndex=ending_row_index(1)  ColSpan=Range of columns  ColStartMode=Index  ColStartIndex=starting_column_index(1)  ColEndMode=Index  ColEndIndex=ending_column_index(1)  DiagSpan=Range of elements  DiagStartMode=Index  DiagStartIndex=2  DiagEndMode=Index  DiagEndIndex=4
  Overwrite Values79 : dspmtrx3/Overwrite Values  OverWriteDiag=Submatrix  valFrom2ndIP=Second input port  ConstValue=0  RowSpan=Range of rows  RowStartMode=Index  RowStartIndex=starting_row_index(2)  RowEndMode=Index  RowEndIndex=ending_row_index(2)  ColSpan=Range of columns  ColStartMode=Index  ColStartIndex=starting_column_index(1)  ColEndMode=Index  ColEndIndex=ending_column_index(1)  DiagSpan=Range of elements  DiagStartMode=Index  DiagStartIndex=2  DiagEndMode=Index  DiagEndIndex=4
  Overwrite Values80 : dspmtrx3/Overwrite Values  OverWriteDiag=Submatrix  valFrom2ndIP=Second input port  ConstValue=0  RowSpan=Range of rows  RowStartMode=Index  RowStartIndex=starting_row_index(4)  RowEndMode=Index  RowEndIndex=ending_row_index(4)  ColSpan=Range of columns  ColStartMode=Index  ColStartIndex=starting_column_index(2)  ColEndMode=Index  ColEndIndex=ending_column_index(2)  DiagSpan=Range of elements  DiagStartMode=Index  DiagStartIndex=2  DiagEndMode=Index  DiagEndIndex=4
  Transpose2 : dspmtrx3/Transpose  Hermitian=off  overflowFlag=off
  wires:
  Demux73/3 -> Matrix Concatenate73/3
  Demux73/5 -> Matrix Concatenate73/5
  Demux73/4 -> Matrix Concatenate73/4
  Demux77/6 -> Matrix Concatenate66/6
  Integer to Bit Converter77/1 -> Demux77/1
  Demux77/5 -> Matrix Concatenate66/5
  Demux77/7 -> Matrix Concatenate66/7
  Demux73/1 -> Matrix Concatenate73/1
  Demux77/4 -> Matrix Concatenate66/4
  Demux73/2 -> Matrix Concatenate73/2
  Demux66/3 -> Matrix Concatenate76/3
  Demux78/7 -> Matrix Concatenate78/7
  Demux75/6 -> Matrix Concatenate74/6
  Demux75/7 -> Matrix Concatenate74/7
  Integer to Bit Converter78/1 -> Demux78/1
  Row7_Col1(8x1B)/1 -> Integer to Bit Converter75/1
  Demux75/2 -> Matrix Concatenate74/2
  Demux76/1 -> Matrix Concatenate77/1
  Demux75/1 -> Matrix Concatenate74/1
  Integer to Bit Converter74/1 -> Demux75/1
  Demux74/1 -> Matrix Concatenate75/1
  Row7_Col3(8x1B)/1 -> Integer to Bit Converter76/1
  Demux74/2 -> Matrix Concatenate75/2
  Integer to Bit Converter75/1 -> Demux74/1
  Demux78/8 -> Matrix Concatenate78/8
  Row7_Col4(8x1B)/1 -> Integer to Bit Converter78/1
  Demux78/1 -> Matrix Concatenate78/1
  Demux78/3 -> Matrix Concatenate78/3
  Demux68/8 -> Matrix Concatenate69/8
  Demux76/7 -> Matrix Concatenate77/7
  Demux78/5 -> Matrix Concatenate78/5
  Integer to Bit Converter76/1 -> Demux76/1
  Row8_Col3(8x1B)/1 -> Integer to Bit Converter70/1
  Demux78/2 -> Matrix Concatenate78/2
  Demux78/4 -> Matrix Concatenate78/4
  Demux75/8 -> Matrix Concatenate74/8
  Demux76/3 -> Matrix Concatenate77/3
  Demux74/4 -> Matrix Concatenate75/4
  Demux74/5 -> Matrix Concatenate75/5
  Row8_Col1(8x1B)/1 -> Integer to Bit Converter69/1
  Demux76/2 -> Matrix Concatenate77/2
  Demux78/6 -> Matrix Concatenate78/6
  Demux68/6 -> Matrix Concatenate69/6
  Demux76/4 -> Matrix Concatenate77/4
  Demux75/5 -> Matrix Concatenate74/5
  Row8_Col4(8x1B)/1 -> Integer to Bit Converter71/1
  Demux74/3 -> Matrix Concatenate75/3
  Demux68/7 -> Matrix Concatenate69/7
  Demux75/3 -> Matrix Concatenate74/3
  Demux75/4 -> Matrix Concatenate74/4
  Demux74/7 -> Matrix Concatenate75/7
  Row8_Col2(8x1B)/1 -> Integer to Bit Converter68/1
  Demux76/8 -> Matrix Concatenate77/8
  Row7_Col2(8x1B)/1 -> Integer to Bit Converter74/1
  Demux68/5 -> Matrix Concatenate69/5
  Integer to Bit Converter69/1 -> Demux68/1
  Demux76/6 -> Matrix Concatenate77/6
  Demux74/6 -> Matrix Concatenate75/6
  Demux76/5 -> Matrix Concatenate77/5
  Demux74/8 -> Matrix Concatenate75/8
  Demux70/1 -> Matrix Concatenate70/1
  Demux70/2 -> Matrix Concatenate70/2
  Demux71/4 -> Matrix Concatenate72/4
  Demux79/6 -> Matrix Concatenate64/6
  Demux79/4 -> Matrix Concatenate64/4
  Demux65/5 -> Matrix Concatenate65/5
  Integer to Bit Converter70/1 -> Demux70/1
  Demux70/5 -> Matrix Concatenate70/5
  Demux70/6 -> Matrix Concatenate70/6
  Demux68/2 -> Matrix Concatenate69/2
  Demux79/3 -> Matrix Concatenate64/3
  Demux69/6 -> Matrix Concatenate68/6
  Demux69/7 -> Matrix Concatenate68/7
  Demux69/5 -> Matrix Concatenate68/5
  Integer to Bit Converter68/1 -> Demux69/1
  Demux69/1 -> Matrix Concatenate68/1
  Demux71/7 -> Matrix Concatenate72/7
  Demux70/7 -> Matrix Concatenate70/7
  Demux68/1 -> Matrix Concatenate69/1
  Demux68/4 -> Matrix Concatenate69/4
  Demux69/4 -> Matrix Concatenate68/4
  Demux70/4 -> Matrix Concatenate70/4
  Demux80/1 -> Matrix Concatenate79/1
  Integer to Bit Converter71/1 -> Demux71/1
  Demux68/3 -> Matrix Concatenate69/3
  Demux69/2 -> Matrix Concatenate68/2
  Demux69/3 -> Matrix Concatenate68/3
  Demux70/3 -> Matrix Concatenate70/3
  Demux71/6 -> Matrix Concatenate72/6
  Demux72/3 -> Matrix Concatenate80/3
  Row8_Col8(8x1B)/1 -> Integer to Bit Converter66/1
  Demux71/5 -> Matrix Concatenate72/5
  Demux73/6 -> Matrix Concatenate73/6
  Demux69/8 -> Matrix Concatenate68/8
  Demux67/1 -> Matrix Concatenate67/1
  Demux77/8 -> Matrix Concatenate66/8
  Integer to Bit Converter73/1 -> Demux72/1
  Demux72/4 -> Matrix Concatenate80/4
  Row8_Col5(8x1B)/1 -> Integer to Bit Converter73/1
  Demux71/2 -> Matrix Concatenate72/2
  Demux71/3 -> Matrix Concatenate72/3
  Demux67/8 -> Matrix Concatenate67/8
  Demux72/2 -> Matrix Concatenate80/2
  Row8_Col7(8x1B)/1 -> Integer to Bit Converter77/1
  Demux72/6 -> Matrix Concatenate80/6
  Row8_Col6(8x1B)/1 -> Integer to Bit Converter72/1
  Demux71/8 -> Matrix Concatenate72/8
  Integer to Bit Converter72/1 -> Demux73/1
  Demux67/6 -> Matrix Concatenate67/6
  Demux72/5 -> Matrix Concatenate80/5
  Demux73/7 -> Matrix Concatenate73/7
  Demux72/7 -> Matrix Concatenate80/7
  Integer to Bit Converter66/1 -> Demux67/1
  Demux72/1 -> Matrix Concatenate80/1
  Demux77/3 -> Matrix Concatenate66/3
  Demux71/1 -> Matrix Concatenate72/1
  Demux73/8 -> Matrix Concatenate73/8
  Demux70/8 -> Matrix Concatenate70/8
  Demux77/2 -> Matrix Concatenate66/2
  Demux72/8 -> Matrix Concatenate80/8
  Demux67/5 -> Matrix Concatenate67/5
  Demux67/3 -> Matrix Concatenate67/3
  Demux67/4 -> Matrix Concatenate67/4
  Demux67/7 -> Matrix Concatenate67/7
  Demux77/1 -> Matrix Concatenate66/1
  Demux67/2 -> Matrix Concatenate67/2
  Demux28/4 -> Matrix Concatenate28/4
  Demux27/3 -> Matrix Concatenate29/3
  Demux30/1 -> Matrix Concatenate31/1
  Demux27/1 -> Matrix Concatenate29/1
  Integer to Bit Converter29/1 -> Demux29/1
  Demux30/6 -> Matrix Concatenate31/6
  Demux28/6 -> Matrix Concatenate28/6
  Demux28/2 -> Matrix Concatenate28/2
  Demux30/8 -> Matrix Concatenate31/8
  Demux30/5 -> Matrix Concatenate31/5
  Overwrite Values69/1 -> Overwrite Values27/1
  Demux28/7 -> Matrix Concatenate28/7
  Demux30/4 -> Matrix Concatenate31/4
  Demux27/4 -> Matrix Concatenate29/4
  Row1_Col2(8x1B)/1 -> Integer to Bit Converter27/1
  Demux30/7 -> Matrix Concatenate31/7
  Row1_Col4(8x1B)/1 -> Integer to Bit Converter30/1
  Demux30/3 -> Matrix Concatenate31/3
  Demux27/6 -> Matrix Concatenate29/6
  Constant1/1 -> Overwrite Values78/1
  Demux28/1 -> Matrix Concatenate28/1
  Overwrite Values29/1 -> Overwrite Values44/1
  Demux27/7 -> Matrix Concatenate29/7
  Demux27/5 -> Matrix Concatenate29/5
  Demux27/8 -> Matrix Concatenate29/8
  Demux28/8 -> Matrix Concatenate28/8
  Row1_Col3(8x1B)/1 -> Integer to Bit Converter29/1
  Overwrite Values71/1 -> Overwrite Values42/1
  Demux30/2 -> Matrix Concatenate31/2
  Demux28/5 -> Matrix Concatenate28/5
  Integer to Bit Converter27/1 -> Demux28/1
  Demux29/8 -> Matrix Concatenate30/8
  Demux28/3 -> Matrix Concatenate28/3
  Overwrite Values77/1 -> Overwrite Values17/1
  Transpose2/1 -> Matrix Viewer3/1
  Overwrite Values76/1 -> Overwrite Values79/1
  Overwrite Values70/1 -> Overwrite Values33/1
  Overwrite Values74/1 -> Overwrite Values46/1
  Demux50/1 -> Matrix Concatenate60/1
  Integer to Bit Converter51/1 -> Demux50/1
  Row5_Col5(8x1B)/1 -> Integer to Bit Converter64/1
  Demux63/7 -> Matrix Concatenate49/7
  Row5_Col8(8x1B)/1 -> Integer to Bit Converter51/1
  Demux50/6 -> Matrix Concatenate60/6
  Demux63/6 -> Matrix Concatenate49/6
  Demux64/6 -> Matrix Concatenate63/6
  Demux49/4 -> Matrix Concatenate50/4
  Demux64/4 -> Matrix Concatenate63/4
  Demux64/3 -> Matrix Concatenate63/3
  Integer to Bit Converter64/1 -> Demux63/1
  Demux50/3 -> Matrix Concatenate60/3
  Demux64/8 -> Matrix Concatenate63/8
  Demux49/1 -> Matrix Concatenate50/1
  Integer to Bit Converter49/1 -> Demux49/1
  Demux53/6 -> Matrix Concatenate53/6
  Demux63/5 -> Matrix Concatenate49/5
  Demux49/5 -> Matrix Concatenate50/5
  Demux64/5 -> Matrix Concatenate63/5
  Demux52/1 -> Matrix Concatenate54/1
  Demux61/1 -> Matrix Concatenate51/1
  Demux50/5 -> Matrix Concatenate60/5
  Row6_Col6(8x1B)/1 -> Integer to Bit Converter56/1
  Demux52/7 -> Matrix Concatenate54/7
  Demux56/7 -> Matrix Concatenate71/7
  Row6_Col7(8x1B)/1 -> Integer to Bit Converter61/1
  Demux57/1 -> Matrix Concatenate57/1
  Demux53/8 -> Matrix Concatenate53/8
  Demux54/4 -> Matrix Concatenate55/4
  Demux53/3 -> Matrix Concatenate53/3
  Demux59/6 -> Matrix Concatenate58/6
  Demux53/4 -> Matrix Concatenate53/4
  Demux55/5 -> Matrix Concatenate56/5
  Demux53/2 -> Matrix Concatenate53/2
  Demux58/8 -> Matrix Concatenate59/8
  Demux51/1 -> Matrix Concatenate52/1
  Demux59/4 -> Matrix Concatenate58/4
  Integer to Bit Converter63/1 -> Demux64/1
  Demux63/8 -> Matrix Concatenate49/8
  Demux52/3 -> Matrix Concatenate54/3
  Demux54/8 -> Matrix Concatenate55/8
  Demux53/7 -> Matrix Concatenate53/7
  Demux62/4 -> Matrix Concatenate62/4
  Row5_Col2(8x1B)/1 -> Integer to Bit Converter58/1
  Demux58/2 -> Matrix Concatenate59/2
  Demux55/6 -> Matrix Concatenate56/6
  Demux52/4 -> Matrix Concatenate54/4
  Demux56/6 -> Matrix Concatenate71/6
  Demux65/6 -> Matrix Concatenate65/6
  Demux58/5 -> Matrix Concatenate59/5
  Demux50/4 -> Matrix Concatenate60/4
  Demux49/8 -> Matrix Concatenate50/8
  Demux50/7 -> Matrix Concatenate60/7
  Demux64/2 -> Matrix Concatenate63/2
  Demux64/1 -> Matrix Concatenate63/1
  Demux64/7 -> Matrix Concatenate63/7
  Demux55/7 -> Matrix Concatenate56/7
  Demux55/2 -> Matrix Concatenate56/2
  Demux54/3 -> Matrix Concatenate55/3
  Demux55/1 -> Matrix Concatenate56/1
  Integer to Bit Converter55/1 -> Demux55/1
  Demux54/2 -> Matrix Concatenate55/2
  Demux55/3 -> Matrix Concatenate56/3
  Demux54/6 -> Matrix Concatenate55/6
  Demux54/7 -> Matrix Concatenate55/7
  Demux53/5 -> Matrix Concatenate53/5
  Demux54/1 -> Matrix Concatenate55/1
  Demux57/6 -> Matrix Concatenate57/6
  Demux51/8 -> Matrix Concatenate52/8
  Demux51/2 -> Matrix Concatenate52/2
  Demux51/6 -> Matrix Concatenate52/6
  Integer to Bit Converter54/1 -> Demux54/1
  Demux61/2 -> Matrix Concatenate51/2
  Demux60/2 -> Matrix Concatenate61/2
  Demux61/3 -> Matrix Concatenate51/3
  Demux62/2 -> Matrix Concatenate62/2
  Demux52/2 -> Matrix Concatenate54/2
  Demux63/3 -> Matrix Concatenate49/3
  Demux63/4 -> Matrix Concatenate49/4
  Demux61/4 -> Matrix Concatenate51/4
  Demux56/8 -> Matrix Concatenate71/8
  Row6_Col2(8x1B)/1 -> Integer to Bit Converter52/1
  Demux60/4 -> Matrix Concatenate61/4
  Integer to Bit Converter53/1 -> Demux52/1
  Integer to Bit Converter62/1 -> Demux62/1
  Demux51/7 -> Matrix Concatenate52/7
  Demux56/5 -> Matrix Concatenate71/5
  Demux49/6 -> Matrix Concatenate50/6
  Integer to Bit Converter50/1 -> Demux51/1
  Demux62/5 -> Matrix Concatenate62/5
  Demux61/8 -> Matrix Concatenate51/8
  Row7_Col8(8x1B)/1 -> Integer to Bit Converter67/1
  Demux59/7 -> Matrix Concatenate58/7
  Demux66/4 -> Matrix Concatenate76/4
  Row6_Col3(8x1B)/1 -> Integer to Bit Converter54/1
  Demux51/4 -> Matrix Concatenate52/4
  Integer to Bit Converter60/1 -> Demux60/1
  Demux58/1 -> Matrix Concatenate59/1
  Row5_Col1(8x1B)/1 -> Integer to Bit Converter59/1
  Demux56/3 -> Matrix Concatenate71/3
  Demux57/8 -> Matrix Concatenate57/8
  Integer to Bit Converter58/1 -> Demux59/1
  Demux56/4 -> Matrix Concatenate71/4
  Integer to Bit Converter57/1 -> Demux56/1
  Demux59/3 -> Matrix Concatenate58/3
  Demux56/2 -> Matrix Concatenate71/2
  Demux52/8 -> Matrix Concatenate54/8
  Integer to Bit Converter52/1 -> Demux53/1
  Demux55/4 -> Matrix Concatenate56/4
  Demux53/1 -> Matrix Concatenate53/1
  Demux51/3 -> Matrix Concatenate52/3
  Demux60/1 -> Matrix Concatenate61/1
  Integer to Bit Converter67/1 -> Demux66/1
  Demux60/7 -> Matrix Concatenate61/7
  Demux51/5 -> Matrix Concatenate52/5
  Demux61/5 -> Matrix Concatenate51/5
  Integer to Bit Converter59/1 -> Demux58/1
  Demux57/2 -> Matrix Concatenate57/2
  Demux52/6 -> Matrix Concatenate54/6
  Row6_Col5(8x1B)/1 -> Integer to Bit Converter57/1
  Demux79/5 -> Matrix Concatenate64/5
  Demux57/5 -> Matrix Concatenate57/5
  Demux58/7 -> Matrix Concatenate59/7
  Demux54/5 -> Matrix Concatenate55/5
  Demux61/6 -> Matrix Concatenate51/6
  Row6_Col1(8x1B)/1 -> Integer to Bit Converter53/1
  Row5_Col4(8x1B)/1 -> Integer to Bit Converter62/1
  Demux79/2 -> Matrix Concatenate64/2
  Integer to Bit Converter65/1 -> Demux65/1
  Demux80/2 -> Matrix Concatenate79/2
  Demux59/1 -> Matrix Concatenate58/1
  Demux58/4 -> Matrix Concatenate59/4
  Demux79/1 -> Matrix Concatenate64/1
  Demux66/1 -> Matrix Concatenate76/1
  Demux60/3 -> Matrix Concatenate61/3
  Row7_Col5(8x1B)/1 -> Integer to Bit Converter80/1
  Demux59/8 -> Matrix Concatenate58/8
  Demux62/7 -> Matrix Concatenate62/7
  Demux59/2 -> Matrix Concatenate58/2
  Demux49/2 -> Matrix Concatenate50/2
  Row5_Col6(8x1B)/1 -> Integer to Bit Converter63/1
  Demux63/2 -> Matrix Concatenate49/2
  Demux58/6 -> Matrix Concatenate59/6
  Demux80/8 -> Matrix Concatenate79/8
  Demux62/6 -> Matrix Concatenate62/6
  Demux59/5 -> Matrix Concatenate58/5
  Demux66/8 -> Matrix Concatenate76/8
  Demux80/4 -> Matrix Concatenate79/4
  Demux65/7 -> Matrix Concatenate65/7
  Demux66/5 -> Matrix Concatenate76/5
  Demux79/8 -> Matrix Concatenate64/8
  Demux80/5 -> Matrix Concatenate79/5
  Demux60/5 -> Matrix Concatenate61/5
  Demux66/7 -> Matrix Concatenate76/7
  Demux60/6 -> Matrix Concatenate61/6
  Demux58/3 -> Matrix Concatenate59/3
  Row6_Col4(8x1B)/1 -> Integer to Bit Converter55/1
  Demux60/8 -> Matrix Concatenate61/8
  Demux52/5 -> Matrix Concatenate54/5
  Demux66/2 -> Matrix Concatenate76/2
  Demux62/1 -> Matrix Concatenate62/1
  Demux62/8 -> Matrix Concatenate62/8
  Demux65/8 -> Matrix Concatenate65/8
  Demux65/3 -> Matrix Concatenate65/3
  Demux57/7 -> Matrix Concatenate57/7
  Demux79/7 -> Matrix Concatenate64/7
  Demux80/6 -> Matrix Concatenate79/6
  Demux61/7 -> Matrix Concatenate51/7
  Demux55/8 -> Matrix Concatenate56/8
  Integer to Bit Converter61/1 -> Demux61/1
  Row7_Col6(8x1B)/1 -> Integer to Bit Converter79/1
  Demux57/3 -> Matrix Concatenate57/3
  Demux57/4 -> Matrix Concatenate57/4
  Integer to Bit Converter79/1 -> Demux80/1
  Demux65/4 -> Matrix Concatenate65/4
  Integer to Bit Converter80/1 -> Demux79/1
  Demux56/1 -> Matrix Concatenate71/1
  Demux65/2 -> Matrix Concatenate65/2
  Row7_Col7(8x1B)/1 -> Integer to Bit Converter65/1
  Demux66/6 -> Matrix Concatenate76/6
  Demux65/1 -> Matrix Concatenate65/1
  Demux62/3 -> Matrix Concatenate62/3
  Row6_Col8(8x1B)/1 -> Integer to Bit Converter50/1
  Integer to Bit Converter56/1 -> Demux57/1
  Row5_Col3(8x1B)/1 -> Integer to Bit Converter60/1
  Demux80/3 -> Matrix Concatenate79/3
  Demux63/1 -> Matrix Concatenate49/1
  Row5_Col7(8x1B)/1 -> Integer to Bit Converter49/1
  Demux50/8 -> Matrix Concatenate60/8
  Demux80/7 -> Matrix Concatenate79/7
  Demux49/3 -> Matrix Concatenate50/3
  Demux49/7 -> Matrix Concatenate50/7
  Demux50/2 -> Matrix Concatenate60/2
  Integer to Bit Converter30/1 -> Demux30/1
  Demux32/5 -> Matrix Concatenate32/5
  Demux32/1 -> Matrix Concatenate32/1
  Row1_Col6(8x1B)/1 -> Integer to Bit Converter31/1
  Demux32/7 -> Matrix Concatenate32/7
  Demux2/1 -> Matrix Concatenate3/1
  Demux1/4 -> Matrix Concatenate2/4
  Demux32/2 -> Matrix Concatenate32/2
  Demux31/8 -> Matrix Concatenate1/8
  Row1_Col5(8x1B)/1 -> Integer to Bit Converter32/1
  Integer to Bit Converter32/1 -> Demux31/1
  Demux32/4 -> Matrix Concatenate32/4
  Integer to Bit Converter2/1 -> Demux2/1
  Demux1/6 -> Matrix Concatenate2/6
  Demux2/7 -> Matrix Concatenate3/7
  Demux20/2 -> Matrix Concatenate22/2
  Demux26/6 -> Matrix Concatenate27/6
  Demux3/1 -> Matrix Concatenate21/1
  Demux20/7 -> Matrix Concatenate22/7
  Demux20/1 -> Matrix Concatenate22/1
  Demux3/4 -> Matrix Concatenate21/4
  Demux3/2 -> Matrix Concatenate21/2
  Demux3/3 -> Matrix Concatenate21/3
  Demux32/6 -> Matrix Concatenate32/6
  Integer to Bit Converter17/1 -> Demux20/1
  Demux20/5 -> Matrix Concatenate22/5
  Demux20/4 -> Matrix Concatenate22/4
  Demux20/3 -> Matrix Concatenate22/3
  Demux3/8 -> Matrix Concatenate21/8
  Demux20/8 -> Matrix Concatenate22/8
  Demux25/6 -> Matrix Concatenate4/6
  Demux25/3 -> Matrix Concatenate4/3
  Demux22/1 -> Matrix Concatenate23/1
  Row2_Col5(8x1B)/1 -> Integer to Bit Converter26/1
  Integer to Bit Converter26/1 -> Demux25/1
  Demux25/8 -> Matrix Concatenate4/8
  Demux24/3 -> Matrix Concatenate26/3
  Demux24/2 -> Matrix Concatenate26/2
  Demux24/1 -> Matrix Concatenate26/1
  Demux22/8 -> Matrix Concatenate23/8
  Integer to Bit Converter25/1 -> Demux26/1
  Demux24/8 -> Matrix Concatenate26/8
  Row2_Col8(8x1B)/1 -> Integer to Bit Converter17/1
  Row2_Col6(8x1B)/1 -> Integer to Bit Converter25/1
  Row2_Col7(8x1B)/1 -> Integer to Bit Converter3/1
  Demux25/7 -> Matrix Concatenate4/7
  Demux25/5 -> Matrix Concatenate4/5
  Demux25/2 -> Matrix Concatenate4/2
  Demux25/1 -> Matrix Concatenate4/1
  Demux26/7 -> Matrix Concatenate27/7
  Demux22/4 -> Matrix Concatenate23/4
  Demux23/8 -> Matrix Concatenate25/8
  Demux23/4 -> Matrix Concatenate25/4
  Demux23/1 -> Matrix Concatenate25/1
  Demux26/8 -> Matrix Concatenate27/8
  Demux23/7 -> Matrix Concatenate25/7
  Demux21/4 -> Matrix Concatenate24/4
  Demux23/3 -> Matrix Concatenate25/3
  Demux22/6 -> Matrix Concatenate23/6
  Integer to Bit Converter21/1 -> Demux22/1
  Demux24/4 -> Matrix Concatenate26/4
  Demux23/2 -> Matrix Concatenate25/2
  Demux23/5 -> Matrix Concatenate25/5
  Demux22/2 -> Matrix Concatenate23/2
  Demux21/2 -> Matrix Concatenate24/2
  Demux22/5 -> Matrix Concatenate23/5
  Demux24/6 -> Matrix Concatenate26/6
  Demux21/1 -> Matrix Concatenate24/1
  Integer to Bit Converter23/1 -> Demux23/1
  Demux22/3 -> Matrix Concatenate23/3
  Demux21/3 -> Matrix Concatenate24/3
  Integer to Bit Converter24/1 -> Demux24/1
  Demux31/3 -> Matrix Concatenate1/3
  Demux31/4 -> Matrix Concatenate1/4
  Demux23/6 -> Matrix Concatenate25/6
  Demux24/7 -> Matrix Concatenate26/7
  Demux1/3 -> Matrix Concatenate2/3
  Demux2/6 -> Matrix Concatenate3/6
  Demux1/8 -> Matrix Concatenate2/8
  Demux1/2 -> Matrix Concatenate2/2
  Demux32/3 -> Matrix Concatenate32/3
  Demux1/7 -> Matrix Concatenate2/7
  Demux32/8 -> Matrix Concatenate32/8
  Row1_Col7(8x1B)/1 -> Integer to Bit Converter1/1
  Demux1/5 -> Matrix Concatenate2/5
  Demux2/3 -> Matrix Concatenate3/3
  Demux31/6 -> Matrix Concatenate1/6
  Demux2/5 -> Matrix Concatenate3/5
  Demux31/1 -> Matrix Concatenate1/1
  Demux2/8 -> Matrix Concatenate3/8
  Demux1/1 -> Matrix Concatenate2/1
  Demux31/7 -> Matrix Concatenate1/7
  Row1_Col8(8x1B)/1 -> Integer to Bit Converter2/1
  Demux2/2 -> Matrix Concatenate3/2
  Demux2/4 -> Matrix Concatenate3/4
  Demux24/5 -> Matrix Concatenate26/5
  Integer to Bit Converter31/1 -> Demux32/1
  Demux31/5 -> Matrix Concatenate1/5
  Integer to Bit Converter1/1 -> Demux1/1
  Matrix Concatenate4/1 -> Overwrite Values51/2
  Overwrite Values59/1 -> Overwrite Values68/1
  Overwrite Values60/1 -> Overwrite Values69/1
  Overwrite Values66/1 -> Overwrite Values75/1
  Overwrite Values55/1 -> Overwrite Values64/1
  Overwrite Values65/1 -> Overwrite Values74/1
  Matrix Concatenate35/1 -> Overwrite Values62/2
  Matrix Concatenate34/1 -> Overwrite Values60/2
  Matrix Concatenate76/1 -> Overwrite Values74/2
  Matrix Concatenate52/1 -> Overwrite Values73/2
  Matrix Concatenate60/1 -> Overwrite Values71/2
  Matrix Concatenate36/1 -> Overwrite Values70/2
  Matrix Concatenate44/1 -> Overwrite Values69/2
  Overwrite Values40/1 -> Overwrite Values55/1
  Matrix Concatenate66/1 -> Overwrite Values66/2
  Matrix Concatenate65/1 -> Overwrite Values65/2
  Matrix Concatenate51/1 -> Overwrite Values64/2
  Matrix Concatenate50/1 -> Overwrite Values63/2
  Overwrite Values44/1 -> Overwrite Values57/1
  Matrix Concatenate49/1 -> Overwrite Values36/2
  Overwrite Values62/1 -> Overwrite Values70/1
  Overwrite Values63/1 -> Overwrite Values71/1
  Matrix Concatenate67/1 -> Overwrite Values75/2
  Overwrite Values52/1 -> Overwrite Values60/1
  Overwrite Values53/1 -> Overwrite Values62/1
  Overwrite Values54/1 -> Overwrite Values63/1
  Overwrite Values57/1 -> Overwrite Values66/1
  Overwrite Values56/1 -> Overwrite Values65/1
  Matrix Concatenate22/1 -> Overwrite Values77/2
  Matrix Concatenate55/1 -> Overwrite Values61/2
  Overwrite Values42/1 -> Overwrite Values28/1
  Matrix Concatenate78/1 -> Overwrite Values25/2
  Matrix Concatenate56/1 -> Overwrite Values22/2
  Matrix Concatenate80/1 -> Overwrite Values44/2
  Matrix Concatenate64/1 -> Overwrite Values41/2
  Overwrite Values25/1 -> Overwrite Values41/1
  Matrix Concatenate71/1 -> Overwrite Values40/2
  Matrix Concatenate73/1 -> Overwrite Values57/2
  Matrix Concatenate79/1 -> Overwrite Values56/2
  Overwrite Values18/1 -> Overwrite Values50/1
  Overwrite Values41/1 -> Overwrite Values56/1
  Matrix Concatenate54/1 -> Overwrite Values42/2
  Matrix Concatenate63/1 -> Overwrite Values54/2
  Matrix Concatenate41/1 -> Overwrite Values53/2
  Matrix Concatenate47/1 -> Overwrite Values52/2
  Matrix Concatenate27/1 -> Overwrite Values59/2
  Matrix Concatenate72/1 -> Overwrite Values29/2
  Matrix Concatenate77/1 -> Overwrite Values72/2
  Matrix Concatenate70/1 -> Overwrite Values2/2
  Matrix Concatenate74/1 -> Overwrite Values34/2
  Matrix Concatenate68/1 -> Overwrite Values43/2
  Matrix Concatenate69/1 -> Overwrite Values46/2
  Matrix Concatenate75/1 -> Overwrite Values45/2
  Overwrite Values22/1 -> Overwrite Values40/1
  Demux20/6 -> Matrix Concatenate22/6
  Demux22/7 -> Matrix Concatenate23/7
  Demux25/4 -> Matrix Concatenate4/4
  Demux31/2 -> Matrix Concatenate1/2
  Matrix Concatenate24/1 -> Overwrite Values79/2
  Overwrite Values30/1 -> Overwrite Values49/1
  Overwrite Values3/1 -> Overwrite Values30/1
  Matrix Concatenate25/1 -> Overwrite Values4/2
  Matrix Concatenate29/1 -> Overwrite Values78/2
  Overwrite Values75/1 -> Transpose2/1
  Overwrite Values78/1 -> Overwrite Values47/1
  Matrix Concatenate28/1 -> Overwrite Values47/2
  Overwrite Values4/1 -> Overwrite Values31/1
  Overwrite Values80/1 -> Overwrite Values39/1
  Overwrite Values58/1 -> Overwrite Values67/1
  Matrix Concatenate30/1 -> Overwrite Values3/2
  Matrix Concatenate31/1 -> Overwrite Values30/2
  Matrix Concatenate1/1 -> Overwrite Values49/2
  Matrix Concatenate32/1 -> Overwrite Values58/2
  Overwrite Values21/1 -> Overwrite Values36/1
  Matrix Concatenate23/1 -> Overwrite Values48/2
  Overwrite Values79/1 -> Overwrite Values48/1
  Overwrite Values48/1 -> Overwrite Values4/1
  Overwrite Values17/1 -> Overwrite Values1/1
  Overwrite Values1/1 -> Overwrite Values26/1
  Overwrite Values31/1 -> Overwrite Values51/1
  Overwrite Values15/1 -> Overwrite Values32/1
  Overwrite Values27/1 -> Overwrite Values80/1
  Overwrite Values39/1 -> Overwrite Values19/1
  Overwrite Values33/1 -> Overwrite Values18/1
  Overwrite Values50/1 -> Overwrite Values21/1
  Overwrite Values49/1 -> Overwrite Values58/1
  Matrix Concatenate39/1 -> Overwrite Values39/2
  Matrix Concatenate53/1 -> Overwrite Values28/2
  Matrix Concatenate38/1 -> Overwrite Values27/2
  Overwrite Values28/1 -> Overwrite Values61/1
  Overwrite Values51/1 -> Overwrite Values59/1
  Overwrite Values32/1 -> Overwrite Values52/1
  Overwrite Values35/1 -> Overwrite Values53/1
  Overwrite Values36/1 -> Overwrite Values54/1
  Matrix Concatenate33/1 -> Overwrite Values32/2
  Matrix Concatenate26/1 -> Overwrite Values31/2
  Matrix Concatenate46/1 -> Overwrite Values15/2
  Matrix Concatenate45/1 -> Overwrite Values26/2
  Matrix Concatenate42/1 -> Overwrite Values1/2
  Matrix Concatenate43/1 -> Overwrite Values17/2
  Matrix Concatenate2/1 -> Overwrite Values67/2
  Overwrite Values19/1 -> Overwrite Values35/1
  Matrix Concatenate59/1 -> Overwrite Values33/2
  Matrix Concatenate40/1 -> Overwrite Values19/2
  Matrix Concatenate37/1 -> Overwrite Values80/2
  Matrix Concatenate58/1 -> Overwrite Values18/2
  Matrix Concatenate62/1 -> Overwrite Values21/2
  Matrix Concatenate48/1 -> Overwrite Values35/2
  Overwrite Values47/1 -> Overwrite Values3/1
  Demux3/5 -> Matrix Concatenate21/5
  Row2_Col4(8x1B)/1 -> Integer to Bit Converter24/1
  Demux29/1 -> Matrix Concatenate30/1
  Integer to Bit Converter28/1 -> Demux27/1
  Demux29/3 -> Matrix Concatenate30/3
  Integer to Bit Converter22/1 -> Demux21/1
  Demux26/1 -> Matrix Concatenate27/1
  Demux27/2 -> Matrix Concatenate29/2
  Demux21/8 -> Matrix Concatenate24/8
  Overwrite Values26/1 -> Overwrite Values15/1
  Matrix Concatenate21/1 -> Overwrite Values68/2
  Demux21/7 -> Matrix Concatenate24/7
  Matrix Concatenate61/1 -> Overwrite Values50/2
  Matrix Concatenate57/1 -> Overwrite Values55/2
  Demux21/5 -> Matrix Concatenate24/5
  Demux29/2 -> Matrix Concatenate30/2
  Demux26/2 -> Matrix Concatenate27/2
  Demux3/7 -> Matrix Concatenate21/7
  Row2_Col1(8x1B)/1 -> Integer to Bit Converter22/1
  Demux29/5 -> Matrix Concatenate30/5
  Demux3/6 -> Matrix Concatenate21/6
  Row2_Col2(8x1B)/1 -> Integer to Bit Converter21/1
  Demux29/7 -> Matrix Concatenate30/7
  Demux29/6 -> Matrix Concatenate30/6
  Overwrite Values72/1 -> Overwrite Values25/1
  Demux26/5 -> Matrix Concatenate27/5
  Overwrite Values46/1 -> Overwrite Values43/1
  Overwrite Values34/1 -> Overwrite Values72/1
  Overwrite Values43/1 -> Overwrite Values2/1
  Overwrite Values61/1 -> Overwrite Values22/1
  Overwrite Values2/1 -> Overwrite Values29/1
  Overwrite Values64/1 -> Overwrite Values73/1
  Overwrite Values67/1 -> Overwrite Values76/1
  Overwrite Values45/1 -> Overwrite Values34/1
  Matrix Concatenate3/1 -> Overwrite Values76/2
  Overwrite Values68/1 -> Overwrite Values77/1
  Demux29/4 -> Matrix Concatenate30/4
  Demux26/3 -> Matrix Concatenate27/3
  Demux21/6 -> Matrix Concatenate24/6
  Row2_Col3(8x1B)/1 -> Integer to Bit Converter23/1
  Demux26/4 -> Matrix Concatenate27/4
  Integer to Bit Converter3/1 -> Demux3/1
  Row1_Col1(8x1B)/1 -> Integer to Bit Converter28/1
  Demux47/8 -> Matrix Concatenate33/8
  Row3_Col5(8x1B)/1 -> Integer to Bit Converter48/1
  Integer to Bit Converter48/1 -> Demux47/1
  Demux48/4 -> Matrix Concatenate47/4
  Integer to Bit Converter35/1 -> Demux34/1
  Demux33/6 -> Matrix Concatenate34/6
  Row3_Col6(8x1B)/1 -> Integer to Bit Converter47/1
  Demux48/7 -> Matrix Concatenate47/7
  Demux34/1 -> Matrix Concatenate44/1
  Demux33/4 -> Matrix Concatenate34/4
  Demux48/2 -> Matrix Concatenate47/2
  Demux34/7 -> Matrix Concatenate44/7
  Demux33/8 -> Matrix Concatenate34/8
  Demux34/4 -> Matrix Concatenate44/4
  Demux48/5 -> Matrix Concatenate47/5
  Demux34/2 -> Matrix Concatenate44/2
  Demux34/5 -> Matrix Concatenate44/5
  Demux34/6 -> Matrix Concatenate44/6
  Row3_Col8(8x1B)/1 -> Integer to Bit Converter35/1
  Demux33/3 -> Matrix Concatenate34/3
  Demux47/2 -> Matrix Concatenate33/2
  Demux47/7 -> Matrix Concatenate33/7
  Demux33/1 -> Matrix Concatenate34/1
  Demux48/6 -> Matrix Concatenate47/6
  Row3_Col7(8x1B)/1 -> Integer to Bit Converter33/1
  Demux48/8 -> Matrix Concatenate47/8
  Demux33/7 -> Matrix Concatenate34/7
  Demux48/3 -> Matrix Concatenate47/3
  Demux33/2 -> Matrix Concatenate34/2
  Demux34/8 -> Matrix Concatenate44/8
  Demux47/1 -> Matrix Concatenate33/1
  Integer to Bit Converter47/1 -> Demux48/1
  Demux47/5 -> Matrix Concatenate33/5
  Integer to Bit Converter33/1 -> Demux33/1
  Demux34/3 -> Matrix Concatenate44/3
  Demux33/5 -> Matrix Concatenate34/5
  Demux47/6 -> Matrix Concatenate33/6
  Demux47/4 -> Matrix Concatenate33/4
  Demux47/3 -> Matrix Concatenate33/3
  Demux48/1 -> Matrix Concatenate47/1
  Integer to Bit Converter39/1 -> Demux39/1
  Demux37/2 -> Matrix Concatenate37/2
  Demux36/3 -> Matrix Concatenate38/3
  Demux38/1 -> Matrix Concatenate39/1
  Demux37/3 -> Matrix Concatenate37/3
  Demux37/7 -> Matrix Concatenate37/7
  Demux38/4 -> Matrix Concatenate39/4
  Integer to Bit Converter38/1 -> Demux38/1
  Demux36/1 -> Matrix Concatenate38/1
  Demux37/6 -> Matrix Concatenate37/6
  Demux38/3 -> Matrix Concatenate39/3
  Demux36/4 -> Matrix Concatenate38/4
  Demux38/7 -> Matrix Concatenate39/7
  Demux39/6 -> Matrix Concatenate40/6
  Demux37/5 -> Matrix Concatenate37/5
  Demux36/2 -> Matrix Concatenate38/2
  Demux38/6 -> Matrix Concatenate39/6
  Demux39/7 -> Matrix Concatenate40/7
  Demux38/2 -> Matrix Concatenate39/2
  Demux39/4 -> Matrix Concatenate40/4
  Integer to Bit Converter36/1 -> Demux37/1
  Demux38/5 -> Matrix Concatenate39/5
  Demux37/4 -> Matrix Concatenate37/4
  Demux37/1 -> Matrix Concatenate37/1
  Demux39/5 -> Matrix Concatenate40/5
  Demux41/7 -> Matrix Concatenate41/7
  Integer to Bit Converter40/1 -> Demux41/1
  Demux40/1 -> Matrix Concatenate48/1
  Demux40/2 -> Matrix Concatenate48/2
  Demux40/3 -> Matrix Concatenate48/3
  Demux40/4 -> Matrix Concatenate48/4
  Demux40/5 -> Matrix Concatenate48/5
  Demux40/6 -> Matrix Concatenate48/6
  Demux40/7 -> Matrix Concatenate48/7
  Demux40/8 -> Matrix Concatenate48/8
  Integer to Bit Converter41/1 -> Demux40/1
  Row4_Col5(8x1B)/1 -> Integer to Bit Converter41/1
  Row4_Col7(8x1B)/1 -> Integer to Bit Converter45/1
  Row4_Col6(8x1B)/1 -> Integer to Bit Converter40/1
  Row4_Col8(8x1B)/1 -> Integer to Bit Converter34/1
  Demux39/8 -> Matrix Concatenate40/8
  Demux38/8 -> Matrix Concatenate39/8
  Demux37/8 -> Matrix Concatenate37/8
  Demux39/1 -> Matrix Concatenate40/1
  Demux39/2 -> Matrix Concatenate40/2
  Demux39/3 -> Matrix Concatenate40/3
  Demux41/6 -> Matrix Concatenate41/6
  Demux35/8 -> Matrix Concatenate36/8
  Demux45/8 -> Matrix Concatenate35/8
  Demux41/8 -> Matrix Concatenate41/8
  Demux35/1 -> Matrix Concatenate36/1
  Demux35/2 -> Matrix Concatenate36/2
  Demux35/3 -> Matrix Concatenate36/3
  Demux35/4 -> Matrix Concatenate36/4
  Demux35/5 -> Matrix Concatenate36/5
  Demux35/6 -> Matrix Concatenate36/6
  Demux35/7 -> Matrix Concatenate36/7
  Integer to Bit Converter34/1 -> Demux35/1
  Demux45/1 -> Matrix Concatenate35/1
  Demux45/2 -> Matrix Concatenate35/2
  Demux45/3 -> Matrix Concatenate35/3
  Demux45/4 -> Matrix Concatenate35/4
  Demux45/5 -> Matrix Concatenate35/5
  Demux45/6 -> Matrix Concatenate35/6
  Demux45/7 -> Matrix Concatenate35/7
  Integer to Bit Converter45/1 -> Demux45/1
  Demux41/1 -> Matrix Concatenate41/1
  Demux41/2 -> Matrix Concatenate41/2
  Demux41/3 -> Matrix Concatenate41/3
  Demux41/4 -> Matrix Concatenate41/4
  Demux41/5 -> Matrix Concatenate41/5
  Demux36/6 -> Matrix Concatenate38/6
  Row4_Col1(8x1B)/1 -> Integer to Bit Converter37/1
  Row4_Col3(8x1B)/1 -> Integer to Bit Converter38/1
  Demux36/8 -> Matrix Concatenate38/8
  Row4_Col2(8x1B)/1 -> Integer to Bit Converter36/1
  Demux36/5 -> Matrix Concatenate38/5
  Demux36/7 -> Matrix Concatenate38/7
  Integer to Bit Converter37/1 -> Demux36/1
  Row4_Col4(8x1B)/1 -> Integer to Bit Converter39/1
  Demux44/2 -> Matrix Concatenate45/2
  Demux44/4 -> Matrix Concatenate45/4
  Demux44/3 -> Matrix Concatenate45/3
  Integer to Bit Converter43/1 -> Demux42/1
  Demux44/1 -> Matrix Concatenate45/1
  Demux44/5 -> Matrix Concatenate45/5
  Demux44/6 -> Matrix Concatenate45/6
  Demux44/7 -> Matrix Concatenate45/7
  Demux42/2 -> Matrix Concatenate43/2
  Row3_Col1(8x1B)/1 -> Integer to Bit Converter43/1
  Integer to Bit Converter46/1 -> Demux46/1
  Demux46/4 -> Matrix Concatenate46/4
  Demux42/4 -> Matrix Concatenate43/4
  Integer to Bit Converter44/1 -> Demux44/1
  Demux42/8 -> Matrix Concatenate43/8
  Demux42/1 -> Matrix Concatenate43/1
  Integer to Bit Converter42/1 -> Demux43/1
  Demux42/7 -> Matrix Concatenate43/7
  Demux42/6 -> Matrix Concatenate43/6
  Demux42/5 -> Matrix Concatenate43/5
  Row3_Col2(8x1B)/1 -> Integer to Bit Converter42/1
  Demux43/4 -> Matrix Concatenate42/4
  Demux43/3 -> Matrix Concatenate42/3
  Demux43/6 -> Matrix Concatenate42/6
  Demux43/8 -> Matrix Concatenate42/8
  Demux43/1 -> Matrix Concatenate42/1
  Demux46/7 -> Matrix Concatenate46/7
  Demux43/2 -> Matrix Concatenate42/2
  Demux46/2 -> Matrix Concatenate46/2
  Demux46/3 -> Matrix Concatenate46/3
  Demux46/8 -> Matrix Concatenate46/8
  Demux44/8 -> Matrix Concatenate45/8
  Demux46/5 -> Matrix Concatenate46/5
  Demux46/6 -> Matrix Concatenate46/6
  Demux46/1 -> Matrix Concatenate46/1
  Demux43/5 -> Matrix Concatenate42/5
  Demux42/3 -> Matrix Concatenate43/3
  Demux43/7 -> Matrix Concatenate42/7
  Row3_Col4(8x1B)/1 -> Integer to Bit Converter46/1
  Row3_Col3(8x1B)/1 -> Integer to Bit Converter44/1
  Overwrite Values73/1 -> Overwrite Values45/1
